simulink model "cart_pend_EKF"  (R2019b)
settings: Solver=FixedStepAuto  StartTime=0.0  StopTime=100  FixedStep=0.01  RelTol=1e-3
values from neighbouring files (symbols this model uses):
  A = [0.969169519504925  -0.246386829627017;  0.049277365925403  0.993808202467626]    [DMDc_MW.m]    (also in DMDc_param_sweep.m = real(A); EKF_msd_estimator.m = [0, 1; -k/m, -b/m]; HAVOK.m = AB(:,1:q*m); HAVOK_param_sweep.m = real(A))
  B = [0.049277365925403; 0.001238359506475]    [DMDc_MW.m]    (also in DMDc_param_sweep.m = AB(:,(q*m+1):end); EKF_estimator.m = zeros(nx,1); EKF_msd_estimator.m = [0; 1/m]; HAVOK.m = AB(:,(q*m+1):end))
  C = [0 1]    [DMDc_MW.m]    (also in EKF_estimator.m = eye(6); EKF_msd_estimator.m = [1, 0]; KF_estimator.m = [1, 0]; LS.m)
  D = 0    [DMDc_MW.m]    (also in DMDc_param_sweep.m = (q-1)*Ts; EKF_estimator.m = m*L*L*(M+m*(1-Cx^2)); EKF_msd_estimator.m; HAVOK.m = 3.99)
  f = f_data(k)    [DMDc_MW.m]    (also in EKF_estimator.m = @cartpend; EKF_msd_estimator.m = @msd; HAVOK.m = @nl_msd; LS.m = out.f.Data')
  g = -9.81    [EKF_estimator.m]    (also in cart_pend_EKF_script.m; cart_pend_EKF_setup.m; cart_pend_NLLS.m = 9.81; floating_pendulum_2D.m = -abs(g))
  P0 = 0.01*eye(nx)    [EKF_estimator.m]    (also in EKF_msd_estimator.m = [0.1, 0.1; 0.1, 0.1]; KF_estimator.m = [0, 0; 0, 0]; cart_pend_EKF_script.m = 0.1*eye(nx); cart_pend_EKF_setup.m = 0.5*eye(nx))
  Q = 0.01*eye(nx)    [EKF_estimator.m]    (also in EKF_msd_estimator.m = 0.00000001*eye(nx); KF_estimator.m = B*(sigma_a^2)*B'; cart_pend_EKF_script.m = 0.0000001*eye(nx); cart_pend_EKF_setup.m = diag([0; 0; 0.00001; 0.0000001]))
  R = 0.0001*eye(ny)    [EKF_estimator.m]    (also in EKF_msd_estimator.m = 0.01*eye(ny); KF_estimator.m = 0.01; cart_pend_EKF_script.m = 0.01*eye(ny); cart_pend_EKF_setup.m = 0.001*eye(ny))
  sigma_a = 0.1    [EKF_estimator.m]    (also in EKF_msd_estimator.m; KF_estimator.m; mass_spring_damper_KF_script.m)
  Ts = 0.05    [DMDc_MW.m]    (also in DMDc_param_sweep.m = t(2)-t(1); EKF_msd_estimator.m = 0.01; HAVOK.m = t(2)-t(1); HAVOK_param_sweep.m = t(2)-t(1))
  u0 = 0    [cart_pend_EKF_script.m]    (also in cart_pend_EKF_setup.m; mass_spring_damper_EKF_param_script.m; mass_spring_damper_EKF_script.m; mass_spring_damper_EKF_setup.m)
  x0 = [0; 0; 0; 0; 0; 1]    [EKF_estimator.m]    (also in EKF_msd_estimator.m = [0; 0]; HAVOK.m = [0.5; 0]; KF_estimator.m = [0; 0]; Linear_regression_state_estimator.m = [0;0;0;0])
settings Model: PacingRate=3  Creator=Murray  LastModifiedBy=Murray
settings SolverCC: AlgebraicLoopSolver=LineSearch
settings DebuggingCC: UnderSpecifiedDimensionMsg=warning

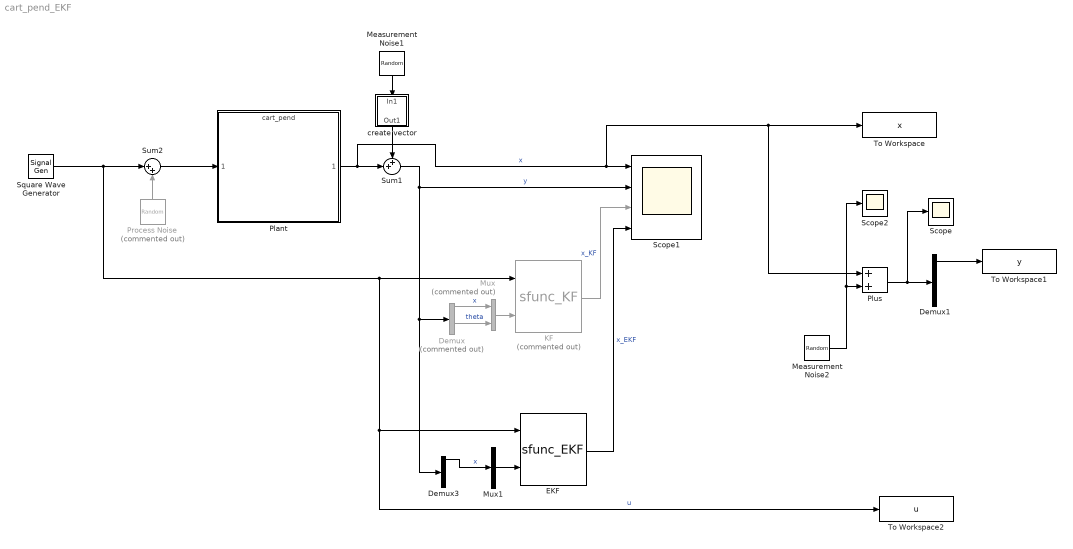
== system cart_pend_EKF ==
  Demux : Demux  Commented=on
  Demux1 : Demux
  Demux3 : Demux
  EKF : M-S-Function  FunctionName=sfunc_EKF  Parameters=Ts,f,g,Q,R,x0,P0,u0
      mask Display:
      | port_label('input', 1, 'u')
      | port_label('input', 2, 'y')
      | port_label('output', 1, 'x_hat')
  KF : M-S-Function  Commented=on  FunctionName=sfunc_KF  Parameters=A,B,C,D,Ts,Q,R,x0,P0
      mask Display:
      | port_label('input', 1, 'u')
      | port_label('input', 2, 'y')
      | port_label('output', 1, 'x_hat')
  Measurement Noise1 : RandomNumber  Variance=R(1,1)  SampleTime=0.01
  Measurement Noise2 : RandomNumber  Variance=R(1,1)  SampleTime=0.01
  Mux : Mux  Commented=on  Inputs=2
  Mux1 : Mux  Inputs=1
  Plant : ModelReference  ModelNameDialog=cart_pend  SimulationMode=Normal  ModelReferenceVersion=1.17
  Plus : Sum
  Process Noise : RandomNumber  Commented=on  Variance=sigma_a^2  SampleTime=0.01
  Scope : Scope
  Scope1 : Scope  NumInputPorts=4
  Scope2 : Scope
  Square Wave Generator : SignalGenerator  WaveForm=square  Amplitude=5  Frequency=1/20
  Sum1 : Sum  Inputs=++|
  Sum2 : Sum  Inputs=|++
  To Workspace : ToWorkspace  VariableName=x  SaveFormat=Timeseries  SampleTime=-1
  To Workspace1 : ToWorkspace  VariableName=y  SaveFormat=Timeseries  SampleTime=-1
  To Workspace2 : ToWorkspace  VariableName=u  SaveFormat=Timeseries  SampleTime=-1
  create vector : Subsystem
  wires:
  Measurement Noise1/1 -> create vector/1(In1)
  create vector/1(Out1) -> Sum1/1
  Plant/1 -> Plus/1, To Workspace/1, Scope1/1, Sum1/2  "x"
  Sum1/1 -> Scope1/2, Demux3/1, Demux/1  "y"
  Process Noise/1 -> Sum2/2
  Sum2/1 -> Plant/1
  KF/1 -> Scope1/3  "x_KF"
  EKF/1 -> Scope1/4  "x_EKF"
  Mux/1 -> KF/2
  Demux/1 -> Mux/1  "x"
  Demux/3 -> Mux/2  "theta"
  Square Wave Generator/1 -> To Workspace2/1, EKF/1, KF/1, Sum2/1  "u"
  Plus/1 -> Demux1/1, Scope/1
  Measurement Noise2/1 -> Scope2/1, Plus/2
  Demux1/1 -> To Workspace1/1
  Mux1/1 -> EKF/2
  Demux3/1 -> Mux1/1  "x"

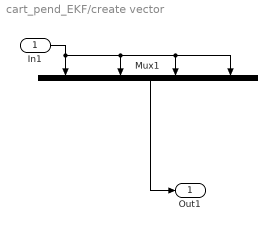
== system cart_pend_EKF/create vector ==
  In1 : Inport
  Mux1 : Mux
  Out1 : Outport
  wires:
  In1/1 -> Mux1/4, Mux1/3, Mux1/2, Mux1/1
  Mux1/1 -> Out1/1
